simulink model "CurrentControl"  (R2022a)
settings: Solver=FixedStepAuto  StartTime=0.0  StopTime=T_end  FixedStep=Ts  RelTol=1e-3
values from neighbouring files (symbols this model uses):
  Cm = 2/m    (= 0.285714285714)    [initializationScript.m]
  K_dec_ax = 1    [initializationScript.m]
  Kid1 = 2*pi*f_b*Rd    (= 150.796447372)    [initializationScript.m]
  Kid3 = 2*pi*f_b*Rd    (= 150.796447372)    [initializationScript.m]
  Kid5 = 2*pi*f_b*Rd    (= 150.796447372)    [initializationScript.m]
  Kiq1 = 2*pi*f_b*Rq    (= 150.796447372)    [initializationScript.m]
  Kiq3 = 2*pi*f_b*Rq    (= 150.796447372)    [initializationScript.m]
  Kiq5 = 2*pi*f_b*Rq    (= 150.796447372)    [initializationScript.m]
  Kpd1 = 2*pi*f_b*Ld    (= 0.314159265359)    [initializationScript.m]
  Kpd3 = 2*pi*f_b*Ld    (= 0.314159265359)    [initializationScript.m]
  Kpd5 = 2*pi*f_b*Ld    (= 0.314159265359)    [initializationScript.m]
  Kpq1 = 2*pi*f_b*Lq    (= 0.314159265359)    [initializationScript.m]
  Kpq3 = 2*pi*f_b*Lq    (= 0.314159265359)    [initializationScript.m]
  Kpq5 = 2*pi*f_b*Lq    (= 0.314159265359)    [initializationScript.m]
  Ld = Ldq    (= 5e-05)    [initializationScript.m]
  Lq = Ldq    (= 5e-05)    [initializationScript.m]
  Lx = Lxy    (= 5e-05)    [initializationScript.m]
  Ly = Lxy    (= 5e-05)    [initializationScript.m]
  Ts = 1/25000    (= 4e-05)    [initializationScript.m]
settings Model: Creator=anvar  LastModifiedBy=Nishanth
settings DataIOCC: SaveOutput=off  SaveTime=off
settings OptimizationCC: DefaultParameterBehavior=Inlined  EnhancedBackFolding=on  PassReuseOutputArgsAs=Individual arguments  ZeroExternalMemoryAtStartup=off  ZeroInternalMemoryAtStartup=off  OptimizeBlockOrder=speed  DifferentSizesBufferReuse=on  OptimizationCustomize=off  EfficientTunableParamExpr=on
settings DebuggingCC: ParameterTunabilityLossMsg=error  UnconnectedInputMsg=warning  UnconnectedOutputMsg=warning  UnconnectedLineMsg=warning
settings SFSimCC: MATLABDynamicMemAlloc=off
settings RTWCC: SystemTargetFile=ert.tlc  TemplateMakefile=ert_default_tmf  DLArmComputeVersion=19.05
settings CodeAppCC: ForceParamTrailComments=on  IgnoreCustomStorageClasses=off  OperatorAnnotations=on  SimulinkDataObjDesc=on  SFDataObjDesc=on  InsertBlockDesc=on
settings ERTTargetCC: TargetLangStandard=C99 (ISO)  GenerateSampleERTMain=on  InlinedParameterPlacement=NonHierarchical  ERTCustomFileTemplate=example_file_process.tlc

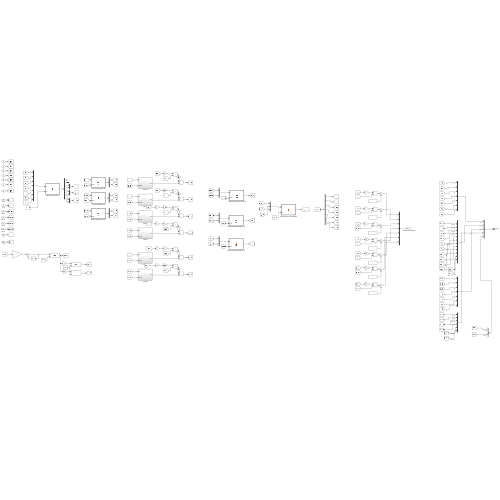
[thumbnail: Simulink's stored preview of the top-level diagram]
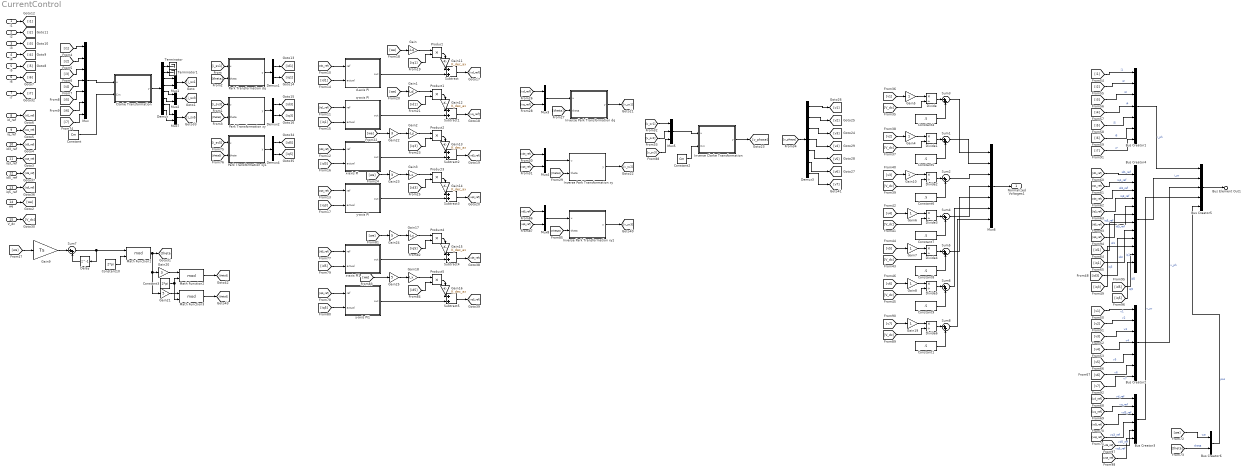
== system CurrentControl ==
  i1 : Inport  OutDataTypeStr=double  PortDimensions=1
  i2 : Inport  Port=2  OutDataTypeStr=double  PortDimensions=1
  i3 : Inport  Port=3  OutDataTypeStr=double  PortDimensions=1
  i4 : Inport  Port=4  OutDataTypeStr=double  PortDimensions=1
  i5 : Inport  Port=5  OutDataTypeStr=double  PortDimensions=1
  i6 : Inport  Port=6  OutDataTypeStr=double  PortDimensions=1
  i7 : Inport  Port=7  OutDataTypeStr=double  PortDimensions=1
  id_ref : Inport  Port=8  OutDataTypeStr=double  PortDimensions=1
  iq_ref : Inport  Port=9  OutDataTypeStr=double  PortDimensions=1
  id3_ref : Inport  Port=10  OutDataTypeStr=double  PortDimensions=1
  iq3_ref : Inport  Port=11  OutDataTypeStr=double  PortDimensions=1
  id5_ref : Inport  Port=12  OutDataTypeStr=double  PortDimensions=1
  iq5_ref : Inport  Port=13  OutDataTypeStr=double  PortDimensions=1
  we : Inport  Port=14  OutDataTypeStr=double  PortDimensions=1
  V_dc : Inport  Port=15  OutDataTypeStr=double  PortDimensions=1
  Bus Creator1 : BusCreator  Inputs=7
  Bus Creator2 : BusCreator  Inputs=7
  Bus Creator3 : BusCreator  Inputs=6
  Bus Creator4 : BusCreator  Inputs=12
  Bus Creator5 : BusCreator  Inputs=5
  Bus Creator6 : BusCreator  Inputs=2
  Clarke Transformation : MATLAB Function  TreatAsAtomicUnit=on
  Constant : Constant  Value=Cm
  Constant{1,4..9} (7 alike) : Constant  Value=.5
  Constant10 : Constant  Value=2*pi
  Constant2 : Constant  Value=Cm
  Constant3 : Constant  Value=2*pi
  Delay : Delay  DelayLength=1
  Demux : Demux  Outputs=8
  Demux1 : Demux  Outputs=2
  Demux2 : Demux  Outputs=2
  Demux3 : Demux  Outputs=7
  Demux4 : Demux  Outputs=2
  Divide{,1..6} (7 alike) : Product  Inputs=*/
  Gain : Gain  Gain=-Lq
  Gain1 : Gain  Gain=Ld
  Gain{4..8,10,19} (7 alike) : Gain
  Gain{11..16} (6 alike) : Gain  Gain=K_dec_ax
  Gain17 : Gain  Gain=-Ly
  Gain18 : Gain  Gain=Lx
  Gain2 : Gain  Gain=-Ly
  Gain20 : Gain  Gain=3
  Gain21 : Gain  Gain=5
  Gain22 : Gain  Gain=3
  Gain23 : Gain  Gain=3
  Gain24 : Gain  Gain=5
  Gain25 : Gain  Gain=5
  Gain3 : Gain  Gain=Lx
  Gain9 : Gain  Gain=Ts
  Inverse Clarke Transformation : MATLAB Function  TreatAsAtomicUnit=on
  Inverse Park Transformation dq : MATLAB Function  TreatAsAtomicUnit=on
  Inverse Park Transformation xy : MATLAB Function  TreatAsAtomicUnit=on
  Inverse Park Transformation xy1 : MATLAB Function  TreatAsAtomicUnit=on
  Math Function1 : Math  Operator=mod  SignedPower=on
  Math Function2 : Math  Operator=mod  SignedPower=on
  Math Function3 : Math  Operator=mod  SignedPower=on
  Mux : Mux  Inputs=7
  Mux{1..4,7..8} (6 alike) : Mux  Inputs=2
  Mux5 : Mux  Inputs=3
  Mux6 : Mux  Inputs=7
  Park Transformation dq : MATLAB Function  TreatAsAtomicUnit=on
  Park Transformation xy : MATLAB Function  TreatAsAtomicUnit=on
  Park Transformation xy1 : MATLAB Function  TreatAsAtomicUnit=on
  Product{,1..5} (6 alike) : Product
  Subtract{,1..5} (6 alike) : Sum
  Sum{1..8} (8 alike) : Sum  Inputs=|++
  Terminator : Terminator
  Terminator1 : Terminator
  d-axis PI : Subsystem
  q-axis PI : Subsystem
  x-axis PI : Subsystem
  x-axis PI1 : Subsystem
  y-axis PI : Subsystem
  y-axis PI1 : Subsystem
  Normalized Voltages1 : Outport
  Bus Element Out1 : Outport  Port=2  PortName=LOG1
  wires:
  Demux3/1 -> [v1]
  [vd3_ref] -> Bus Creator3/3  "vd3_ref"
  Demux3/4 -> [v4]
  [v4] -> Gain6/1
  Sum2/1 -> Mux6/3
  [v1] -> Gain5/1
  Constant8/1 -> Sum5/2
  [V_dc] -> Divide3/2
  Divide4/1 -> Sum5/1
  Constant7/1 -> Sum4/2
  Sum5/1 -> Mux6/5
  Constant9/1 -> Sum6/2
  Gain10/1 -> Divide2/1
  Constant10/1 -> Math Function1/2
  [i3] -> Bus Creator1/3  "i3"
  Sum6/1 -> Mux6/6
  Sum1/1 -> Mux6/2
  [i2] -> Bus Creator1/2  "i2"
  [id1_ref] -> Bus Creator4/1  "id1_ref"
  [iq1_ref] -> Bus Creator4/2  "iq1_ref"
  Bus Creator5/1 -> Bus Element Out1/1
  Bus Creator6/1 -> Bus Creator5/5  "pos"
  [v6] -> Bus Creator2/6  "v6"
  [id3_ref] -> Bus Creator4/3  "id3_ref"
  [V_dc] -> Divide2/2
  [vd_ref] -> Bus Creator3/1  "vd_ref"
  [v2] -> Bus Creator2/2  "v2"
  Bus Creator3/1 -> Bus Creator5/4  "v_sv"
  [vq3_ref] -> Bus Creator3/4  "vq3_ref"
  [we] -> Bus Creator6/1  "we"
  [theta] -> Bus Creator6/2  "theta"
  [iq5] -> y-axis PI1/2(actual)
  Bus Creator1/1 -> Bus Creator5/1  "i_ph"
  Inverse Park Transformation xy1/1(y) -> [v_sv3]
  [v3] -> Bus Creator2/3  "v3"
  [i4] -> Mux/4
  [iq5_ref] -> y-axis PI1/1(ref)
  [we] -> Gain1/1
  Gain17/1 -> Product4/1
  Constant5/1 -> Sum1/2
  y-axis PI1/1(out) -> Subtract5/2
  Demux/1 -> Terminator/1
  [iq3_ref] -> Bus Creator4/4  "iq3_ref"
  [id5_ref] -> x-axis PI1/1(ref)
  Demux4/1 -> [id5]
  Gain16/1 -> Subtract5/1
  Product4/1 -> Gain15/1
  [vq3_ref] -> Mux4/2
  Demux/8 -> Mux7/2
  [theta3] -> Inverse Park Transformation xy/2(theta)
  [v_sv2] -> Mux5/2
  Gain9/1 -> Sum7/1
  Clarke Transformation/1(y) -> Demux/1
  Demux1/1 -> [id1]
  [vq_ref] -> Bus Creator3/2  "vq_ref"
  [i5] -> Mux/5
  Sum7/1 -> Math Function1/1, Delay/1
  Gain14/1 -> Subtract3/1
  Gain11/1 -> Subtract/1
  Delay/1 -> Sum7/2
  Gain13/1 -> Subtract2/1
  Demux2/2 -> [iq3]
  i7/1 -> [i7]
  [iq1] -> q-axis PI/2(actual)
  Constant6/1 -> Sum2/2
  Bus Creator4/1 -> Bus Creator5/2  "i_sv"
  Mux2/1 -> [i_sv3]
  Demux/2 -> Terminator1/1
  Mux/1 -> Clarke Transformation/1(u)
  Bus Creator2/1 -> Bus Creator5/3  "v_ph"
  Demux/3 -> Mux1/1
  Demux/6 -> Mux2/2
  [i_sv1] -> Park Transformation dq/1(u)
  Demux/5 -> Mux2/1
  Subtract1/1 -> [vq_ref]
  [i_sv3] -> Park Transformation xy/1(u)
  we/1 -> [we]
  i2/1 -> [i2]
  [theta] -> Park Transformation dq/2(theta)
  id3_ref/1 -> [id3_ref]
  id_ref/1 -> [id1_ref]
  i4/1 -> [i4]
  Inverse Park Transformation dq/1(y) -> [v_sv1]
  q-axis PI/1(out) -> Subtract1/2
  i3/1 -> [i3]
  i6/1 -> [i6]
  Product1/1 -> Gain12/1
  i5/1 -> [i5]
  [i3] -> Mux/3
  [theta3] -> Park Transformation xy/2(theta)
  [iq1_ref] -> q-axis PI/1(ref)
  Park Transformation xy/1(y) -> Demux2/1
  [id3_ref] -> x-axis PI/1(ref)
  Mux4/1 -> Inverse Park Transformation xy/1(u)
  Mux8/1 -> Inverse Park Transformation xy1/1(u)
  [iq3] -> y-axis PI/2(actual)
  Demux/7 -> Mux7/1
  Demux2/1 -> [id3]
  Divide2/1 -> Sum2/1
  [id1_ref] -> d-axis PI/1(ref)
  [we] -> Gain/1
  Gain1/1 -> Product1/1
  Sum3/1 -> Mux6/1
  [i6] -> Mux/6
  [id1] -> Product1/2
  Product3/1 -> Gain14/1
  Divide5/1 -> Sum6/1
  [v_phase] -> Demux3/1
  x-axis PI/1(out) -> Subtract2/2
  Product/1 -> Gain11/1
  [v2] -> Gain4/1
  [iq3] -> Product2/2
  Gain2/1 -> Product2/1
  [we] -> Gain22/1
  [V_dc] -> Divide/2
  [vq_ref] -> Mux3/2
  Gain7/1 -> Divide4/1
  [vd3_ref] -> Mux4/1
  Constant2/1 -> Inverse Clarke Transformation/2(Cm)
  [V_dc] -> Divide5/2
  [v_sv1] -> Mux5/1
  Subtract/1 -> [vd_ref]
  Gain3/1 -> Product3/1
  Gain8/1 -> Divide5/1
  Constant4/1 -> Sum3/2
  y-axis PI/1(out) -> Subtract3/2
  [we] -> Gain23/1
  [i5] -> Bus Creator1/5  "i5"
  [v_sv3] -> Mux5/3
  Park Transformation xy1/1(y) -> Demux4/1
  [i7] -> Mux/7
  [V_dc] -> Divide4/2
  [iq3_ref] -> y-axis PI/1(ref)
  [vq5_ref] -> Bus Creator3/6  "vq5_ref"
  Mux6/1 -> Normalized Voltages1/1
  Gain25/1 -> Gain18/1
  [v7] -> Gain19/1
  Constant/1 -> Clarke Transformation/2(Cm)
  [v6] -> Gain8/1
  Gain24/1 -> Gain17/1
  Divide1/1 -> Sum1/1
  Gain23/1 -> Gain3/1
  i1/1 -> [i1]
  Gain19/1 -> Divide6/1
  [theta] -> Inverse Park Transformation dq/2(theta)
  [id1] -> d-axis PI/2(actual)
  Constant1/1 -> Sum8/2
  [we] -> Gain9/1
  [vd5_ref] -> Mux8/1
  [v5] -> Bus Creator2/5  "v5"
  Subtract4/1 -> [vd5_ref]
  Gain15/1 -> Subtract4/1
  [v7] -> Bus Creator2/7  "v7"
  Inverse Park Transformation xy/1(y) -> [v_sv2]
  [we] -> Gain24/1
  Math Function2/1 -> [theta3]
  Subtract2/1 -> [vd3_ref]
  Constant3/1 -> Math Function3/2, Math Function2/2
  iq3_ref/1 -> [iq3_ref]
  [i1] -> Mux/1
  [i7] -> Bus Creator1/7  "i7"
  Math Function3/1 -> [theta5]
  iq5_ref/1 -> [iq5_ref]
  [i1] -> Bus Creator1/1  "i1"
  [vq5_ref] -> Mux8/2
  [theta5] -> Park Transformation xy1/2(theta)
  iq_ref/1 -> [iq1_ref]
  [v4] -> Bus Creator2/4  "v4"
  d-axis PI/1(out) -> Subtract/2
  Gain21/1 -> Math Function3/1
  [vd_ref] -> Mux3/1
  [vd5_ref] -> Bus Creator3/5  "vd5_ref"
  Demux/4 -> Mux1/2
  x-axis PI1/1(out) -> Subtract4/2
  Gain20/1 -> Math Function2/1
  id5_ref/1 -> [id5_ref]
  Subtract5/1 -> [vq5_ref]
  [id1] -> Bus Creator4/7  "id1"
  Gain6/1 -> Divide3/1
  [i4] -> Bus Creator1/4  "i4"
  [iq1] -> Product/2
  [id5] -> x-axis PI1/2(actual)
  [id3] -> Bus Creator4/9  "id3"
  Gain5/1 -> Divide/1
  [iq5_ref] -> Bus Creator4/6  "iq5_ref"
  Math Function1/1 -> Gain21/1, Gain20/1, [theta]
  Mux1/1 -> [i_sv1]
  Gain18/1 -> Product5/1
  Demux3/5 -> [v5]
  Demux3/2 -> [v2]
  [we] -> Gain25/1
  [id5_ref] -> Bus Creator4/5  "id5_ref"
  Divide3/1 -> Sum4/1
  [iq5] -> Bus Creator4/12  "iq5"
  [id5] -> Bus Creator4/11  "id5"
  [iq1] -> Bus Creator4/8  "iq1"
  [id3] -> Product3/2
  [V_dc] -> Divide1/2
  Product5/1 -> Gain16/1
  Mux7/1 -> [i_sv5]
  [v5] -> Gain7/1
  Gain4/1 -> Divide1/1
  Gain22/1 -> Gain2/1
  [i_sv5] -> Park Transformation xy1/1(u)
  Sum8/1 -> Mux6/7
  Divide6/1 -> Sum8/1
  [v3] -> Gain10/1
  Gain/1 -> Product/1
  Gain12/1 -> Subtract1/1
  [V_dc] -> Divide6/2
  Mux5/1 -> Inverse Clarke Transformation/1(u)
  Mux3/1 -> Inverse Park Transformation dq/1(u)
  [id3] -> x-axis PI/2(actual)
  [theta5] -> Inverse Park Transformation xy1/2(theta)
  Subtract3/1 -> [vq3_ref]
  Demux3/3 -> [v3]
  Divide/1 -> Sum3/1
  Sum4/1 -> Mux6/4
  Demux3/7 -> [v7]
  [i2] -> Mux/2
  Demux4/2 -> [iq5]
  [i6] -> Bus Creator1/6  "i6"
  [iq5] -> Product4/2
  V_dc/1 -> [V_dc]
  Demux1/2 -> [iq1]
  [id5] -> Product5/2
  [v1] -> Bus Creator2/1  "v1"
  Park Transformation dq/1(y) -> Demux1/1
  Inverse Clarke Transformation/1(y) -> [v_phase]
  Product2/1 -> Gain13/1
  Demux3/6 -> [v6]
  [iq3] -> Bus Creator4/10  "iq3"

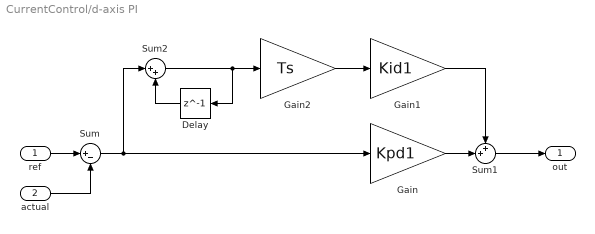
== system CurrentControl/d-axis PI ==
  ref : Inport
  actual : Inport  Port=2
  Delay : Delay  DelayLength=1
  Gain : Gain  Gain=Kpd1
  Gain1 : Gain  Gain=Kid1
  Gain2 : Gain  Gain=Ts
  Sum : Sum  Inputs=|+-
  Sum1 : Sum  Inputs=++|
  Sum2 : Sum  Inputs=|++
  out : Outport
  wires:
  ref/1 -> Sum/1
  Delay/1 -> Sum2/2
  Gain1/1 -> Sum1/1
  Sum/1 -> Gain/1, Sum2/1
  Gain/1 -> Sum1/2
  Gain2/1 -> Gain1/1
  Sum1/1 -> out/1
  actual/1 -> Sum/2
  Sum2/1 -> Delay/1, Gain2/1

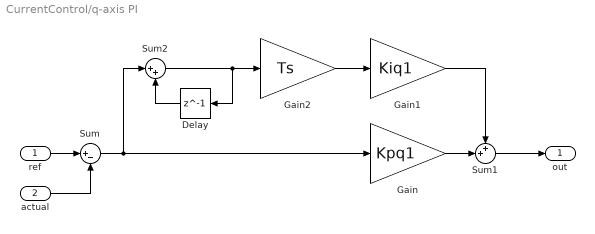
== system CurrentControl/q-axis PI ==
  ref : Inport
  actual : Inport  Port=2
  Delay : Delay  DelayLength=1
  Gain : Gain  Gain=Kpq1
  Gain1 : Gain  Gain=Kiq1
  Gain2 : Gain  Gain=Ts
  Sum : Sum  Inputs=|+-
  Sum1 : Sum  Inputs=++|
  Sum2 : Sum  Inputs=|++
  out : Outport
  wires:
  Sum2/1 -> Gain2/1, Delay/1
  actual/1 -> Sum/2
  Sum1/1 -> out/1
  Gain2/1 -> Gain1/1
  Gain/1 -> Sum1/2
  Sum/1 -> Sum2/1, Gain/1
  Gain1/1 -> Sum1/1
  Delay/1 -> Sum2/2
  ref/1 -> Sum/1

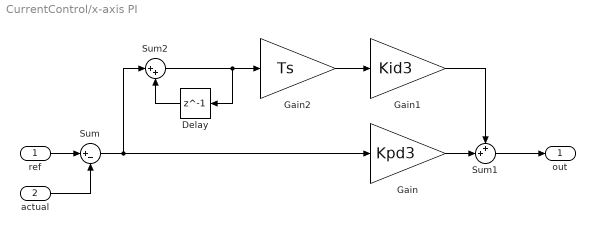
== system CurrentControl/x-axis PI ==
  ref : Inport
  actual : Inport  Port=2
  Delay : Delay  DelayLength=1
  Gain : Gain  Gain=Kpd3
  Gain1 : Gain  Gain=Kid3
  Gain2 : Gain  Gain=Ts
  Sum : Sum  Inputs=|+-
  Sum1 : Sum  Inputs=++|
  Sum2 : Sum  Inputs=|++
  out : Outport
  wires:
  ref/1 -> Sum/1
  Delay/1 -> Sum2/2
  Gain1/1 -> Sum1/1
  Sum/1 -> Gain/1, Sum2/1
  Gain/1 -> Sum1/2
  Gain2/1 -> Gain1/1
  Sum1/1 -> out/1
  actual/1 -> Sum/2
  Sum2/1 -> Delay/1, Gain2/1

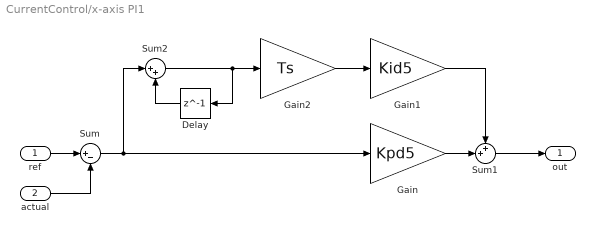
== system CurrentControl/x-axis PI1 ==
  ref : Inport
  actual : Inport  Port=2
  Delay : Delay  DelayLength=1
  Gain : Gain  Gain=Kpd5
  Gain1 : Gain  Gain=Kid5
  Gain2 : Gain  Gain=Ts
  Sum : Sum  Inputs=|+-
  Sum1 : Sum  Inputs=++|
  Sum2 : Sum  Inputs=|++
  out : Outport
  wires:
  Sum2/1 -> Gain2/1, Delay/1
  actual/1 -> Sum/2
  Sum1/1 -> out/1
  Gain2/1 -> Gain1/1
  Gain/1 -> Sum1/2
  Sum/1 -> Sum2/1, Gain/1
  Gain1/1 -> Sum1/1
  Delay/1 -> Sum2/2
  ref/1 -> Sum/1

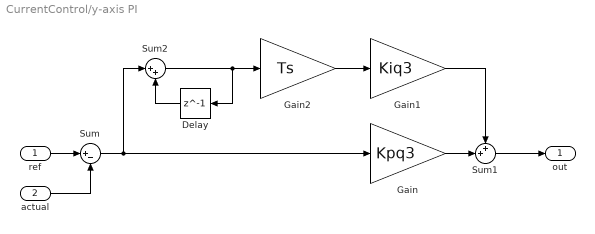
== system CurrentControl/y-axis PI ==
  ref : Inport
  actual : Inport  Port=2
  Delay : Delay  DelayLength=1
  Gain : Gain  Gain=Kpq3
  Gain1 : Gain  Gain=Kiq3
  Gain2 : Gain  Gain=Ts
  Sum : Sum  Inputs=|+-
  Sum1 : Sum  Inputs=++|
  Sum2 : Sum  Inputs=|++
  out : Outport
  wires:
  Sum2/1 -> Gain2/1, Delay/1
  actual/1 -> Sum/2
  Sum1/1 -> out/1
  Gain2/1 -> Gain1/1
  Gain/1 -> Sum1/2
  Sum/1 -> Sum2/1, Gain/1
  Gain1/1 -> Sum1/1
  Delay/1 -> Sum2/2
  ref/1 -> Sum/1

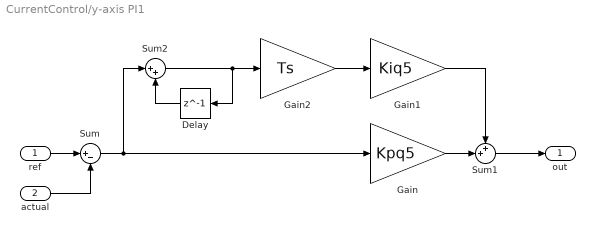
== system CurrentControl/y-axis PI1 ==
  ref : Inport
  actual : Inport  Port=2
  Delay : Delay  DelayLength=1
  Gain : Gain  Gain=Kpq5
  Gain1 : Gain  Gain=Kiq5
  Gain2 : Gain  Gain=Ts
  Sum : Sum  Inputs=|+-
  Sum1 : Sum  Inputs=++|
  Sum2 : Sum  Inputs=|++
  out : Outport
  wires:
  ref/1 -> Sum/1
  Delay/1 -> Sum2/2
  Gain1/1 -> Sum1/1
  Sum/1 -> Gain/1, Sum2/1
  Gain/1 -> Sum1/2
  Gain2/1 -> Gain1/1
  Sum1/1 -> out/1
  actual/1 -> Sum/2
  Sum2/1 -> Delay/1, Gain2/1

== matlab function CurrentControl/Park Transformation dq ==
  data: u input; y output; theta input
function y  = fcn(u,theta)

dq = [cos(theta) sin(theta); -sin(theta) cos(theta)]*u;

d = dq(1);
q = dq(2);
y = [d; q];

== matlab function CurrentControl/Clarke Transformation ==
  data: u input; y output; Cm input
function y = fcn(u,Cm)
m = 7;
length_u = length(u);

x = zeros(m,1);
for i = 1:length_u
    x(i,1) = u(i);
end

if mod(m,2) == 0
    seq_max = m/2 + 1;
else
    seq_max = (m - 1)/2 + 1;
end

Clarke = complex(zeros(seq_max,m));
a = exp(1i*2*pi/m);
for j = 0:seq_max-1
    for i = 1:m
        Clarke(j+1,i) = Cm*a^(j*(i - 1));
    end    
end

vec = Clarke*x;
vec(1,:) = 1/2*vec(1,:);
if mod(m,2) == 0
    vec(m/2+1,:) = 1/2*vec(m/2+1,:);
end

vec1 = [real(vec) imag(vec)];

y = zeros(2*seq_max,1);
y = reshape(vec1',[2*seq_max 1]);

== matlab function CurrentControl/Park Transformation xy ==
  data: u input; y output; theta input
function y  = fcn(u,theta)

dq = [cos(theta) sin(theta); -sin(theta) cos(theta)]*u;

d = dq(1);
q = dq(2);
y = [d; q];

== matlab function CurrentControl/Inverse Park Transformation dq ==
  data: u input; y output; theta input
function y  = fcn(u,theta)

ab = [cos(theta) -sin(theta); sin(theta) cos(theta)]*u;

alpha = ab(1);
beta = ab(2);
y = [alpha; beta];

== matlab function CurrentControl/Inverse Clarke Transformation ==
  data: u input; y output; Cm input
function y = fcn(u,Cm)
m = 7;
Clarke = zeros(6,m);
for i = 1:m
    Clarke(:,i) = Cm*[cos(1*2*pi/m*(i - 1)); sin(1*2*pi/m*(i - 1));...
                      cos(2*2*pi/m*(i - 1)); sin(2*2*pi/m*(i - 1));
                      cos(3*2*pi/m*(i - 1)); sin(3*2*pi/m*(i - 1))];
end

invClarke = pinv(Clarke);

y = invClarke*u;

== matlab function CurrentControl/Inverse Park Transformation xy ==
  data: u input; y output; theta input
function y  = fcn(u,theta)

ab = [cos(theta) -sin(theta); sin(theta) cos(theta)]*u;

alpha = ab(1);
beta = ab(2);
y = [alpha; beta];

== matlab function CurrentControl/Park Transformation xy1 ==
  data: u input; y output; theta input
function y  = fcn(u,theta)

dq = [cos(theta) sin(theta); -sin(theta) cos(theta)]*u;

d = dq(1);
q = dq(2);
y = [d; q];

== matlab function CurrentControl/Inverse Park Transformation xy1 ==
  data: u input; y output; theta input
function y  = fcn(u,theta)

ab = [cos(theta) -sin(theta); sin(theta) cos(theta)]*u;

alpha = ab(1);
beta = ab(2);
y = [alpha; beta];
